simulink model "step_responses_sin"  (R2016b)
settings: Solver=VariableStepAuto  StartTime=0.0  StopTime=10.0  RelTol=1e-3
undefined symbols (not defined in the file): den, num, ts
settings Model: Creator=AdrianCortez  LastModifiedBy=AdrianCortez
settings DataIOCC: ReturnWorkspaceOutputs=on
settings DebuggingCC: UnconnectedInputMsg=none  UnconnectedOutputMsg=none  UnconnectedLineMsg=none
settings ModelReferenceCC: EnableRefExpFcnMdlSchedulingChecks=off
settings SFSimCC: SimUseLocalCustomCode=on
settings RTWCC: RTWUseLocalCustomCode=on

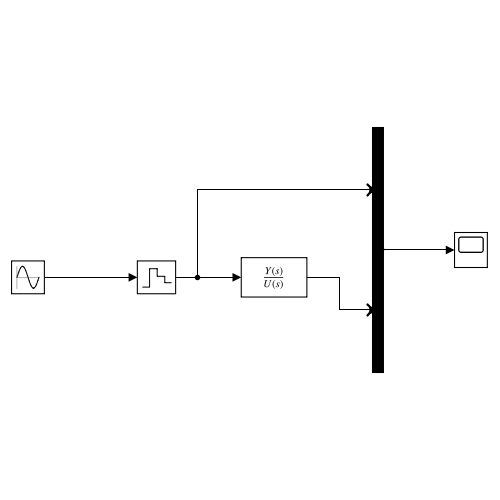
[thumbnail: Simulink's stored preview of the top-level diagram]
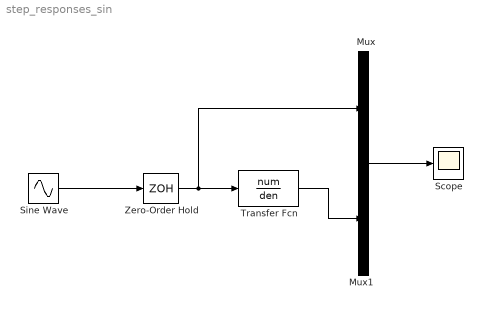
== system step_responses_sin ==
  Mux : Mux  Inputs=2
  Mux1 : Mux  Inputs=2
  Scope : Scope
  Sine Wave : Sin  Frequency=2*pi*1000  SampleTime=0
  Transfer Fcn : TransferFcn  Numerator=num  Denominator=den
  Zero-Order Hold : ZeroOrderHold  SampleTime=ts
  wires:
  Transfer Fcn/1 -> Mux/2
  Mux/1 -> Scope/1
  Sine Wave/1 -> Zero-Order Hold/1
  Zero-Order Hold/1 -> Mux/1, Transfer Fcn/1
